simulink model "AEB_Final_PID"  (R2024b)
settings: Solver=VariableStepAuto  StartTime=0.0  StopTime=4  RelTol=1e-3
libraries: slpidlib x1, simulink x1
settings Model: Creator=garvi  LastModifiedBy=garvi
settings SolverCC: ZeroCrossControl=DisableAll

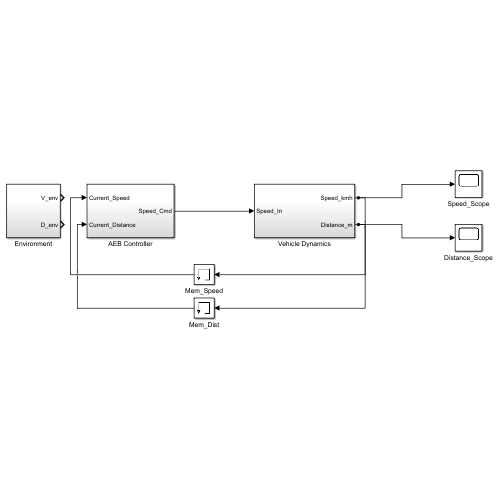
[thumbnail: Simulink's stored preview of the top-level diagram]
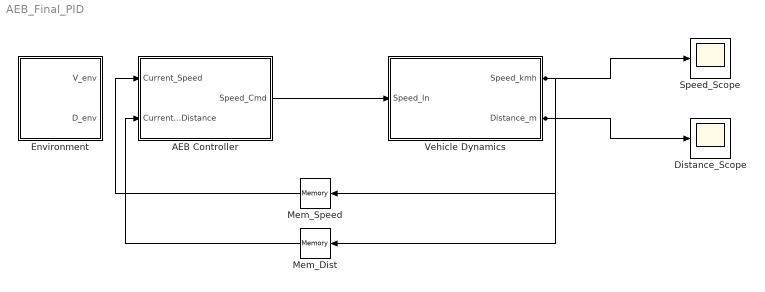
== system AEB_Final_PID ==
  AEB Controller : Subsystem
  Distance_Scope : Scope
  Environment : Subsystem
  Mem_Dist : Memory
  Mem_Speed : Memory
  Speed_Scope : Scope
  Vehicle Dynamics : Subsystem
  wires:
  AEB Controller/1(Speed_Cmd) -> Vehicle Dynamics/1(Speed_In)
  Vehicle Dynamics/1(Speed_kmh) -> Speed_Scope/1, Mem_Speed/1
  Vehicle Dynamics/2(Distance_m) -> Distance_Scope/1, Mem_Dist/1
  Mem_Speed/1 -> AEB Controller/1(Current_Speed)
  Mem_Dist/1 -> AEB Controller/2(Current_Distance)

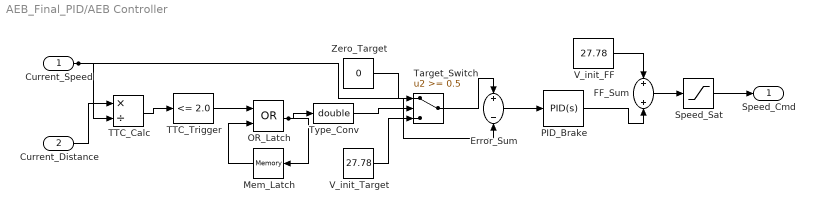
== system AEB_Final_PID/AEB Controller ==
  Current_Speed : Inport
  Current_Distance : Inport  Port=2
  Error_Sum : Sum  Inputs=+-
  FF_Sum : Sum
  Mem_Latch : Memory
  OR_Latch : Logic  Operator=OR  AllPortsSameDT=off  OutDataTypeStr=boolean
  PID_Brake : slpidlib/PID Controller  Controller=PID  Form=Parallel  TimeDomain=Continuous-time  UseExternalTs=off  SampleTime=-1  IntegratorMethod=Forward Euler  FilterMethod=Forward Euler  ControllerParametersSource=internal  P=0.1  I=0.8  UseKiTs=off  D=0  UseExternalDerivativeSource=off  N=100  UseFilter=on  TunerSelectOption=Transfer Function Based (PID Tuner App)  InitialConditionSource=internal  InitialConditionForIntegrator=0  InitialConditionForFilter=0  DifferentiatorICPrevScaledInput=0  ExternalReset=none  TrackingMode=off  Kt=1  LimitOutput=off  SatLimitsSource=internal  UpperSaturationLimit=inf  LowerSaturationLimit=-inf  LinearizeAsGain=on  AntiWindupMode=none  Kb=1  LimitIntegrator=off  UpperIntegratorSaturationLimit=inf  LowerIntegratorSaturationLimit=-inf  POutMin=[]  POutMax=[]  IOutMin=[]  IOutMax=[]  DOutMin=[]  DOutMax=[]  NOutMin=[]  NOutMax=[]  SumOutMin=[]  SumOutMax=[]  SaturationOutMin=[]  SaturationOutMax=[]  PParamMin=[]  PParamMax=[]  IParamMin=[]  IParamMax=[]  DParamMin=[]  DParamMax=[]  NParamMin=[]  NParamMax=[]  KbParamMin=[]  KbParamMax=[]  KtParamMin=[]  KtParamMax=[]  KbOutMin=[]  KbOutMax=[]  KtOutMin=[]  KtOutMax=[]  IntegratorOutMin=[]  IntegratorOutMax=[]  FilterOutMin=[]  FilterOutMax=[]  SumI1OutMin=[]  SumI1OutMax=[]  SumI2OutMin=[]  SumI2OutMax=[]  SumI3OutMin=[]  SumI3OutMax=[]  SumI4OutMin=[]  SumI4OutMax=[]  SumDOutMin=[]  SumDOutMax=[]  DifferentiatorOutMin=[]  DifferentiatorOutMax=[]  FilterDiffOutCoefMin=[]  FilterDiffOutCoefMax=[]  ReciprocalOutMin=[]  ReciprocalOutMax=[]  SumDenOutMin=[]  SumDenOutMax=[]  SumNumOutMin=[]  SumNumOutMax=[]  DivideOutMin=[]  DivideOutMax=[]  UdiffTsProdOutMin=[]  UdiffTsProdOutMax=[]  NTsProdOutMin=[]  NTsProdOutMax=[]  UintegralTsProdOutMin=[]  UintegralTsProdOutMax=[]  UngainTsProdOutMin=[]  UngainTsProdOutMax=[]  ClampingZeroOutDataTypeStr=Inherit: Inherit via back propagation  ClampingZeroOutMin=[]  ClampingZeroOutMax=[]  FilterDenConstantOutDataTypeStr=Inherit: Inherit via back propagation  FilterDenConstantOutMin=[]  FilterDenConstantOutMax=[]  PCopyOutDataTypeStr=Inherit: Inherit via back propagation  PCopyOutMin=[]  PCopyOutMax=[]  NCopyOutDataTypeStr=Inherit: Inherit via back propagation  NCopyOutMin=[]  NCopyOutMax=[]  IntegratorContinuousStateAttributes=''  IntegratorStateMustResolveToSignalObject=off  IntegratorRTWStateStorageClass=Auto  FilterContinuousStateAttributes=''  FilterStateMustResolveToSignalObject=off  FilterRTWStateStorageClass=Auto  ParallelPVariant=InternalParameters  IdealPVariant=Disabled  IVariant=InternalParameters  DVariant=InternalParameters  IntegratorVariant=Continuous  SatVariant=Disabled  AWVariant=Passthrough  PCopyVariant=Disabled  TRVariant=Disabled  FdbkBlocksVariant=Forward  IdealPFdbkVariant=Disabled  SatFdbkVariant=Disabled  DerivativeFilterVariant=ContFilter  NVariant=InternalParameters  NCopyVariant=Disabled  FilterICVariant=InternalICsFilter  IntegratorICVariant=InternalICs  ExternalResetVariant=Disabled  TRSumVariant=Passthrough  SumFdbkVariant=Disabled  SumVariant=Sum_PID  TsampFilterVariant=InternalTs  TsampNgainVariant=Passthrough  TsampIntegralVariant=Disabled_SignalSpec  ExternalSaturationOutDataTypeStr=Inherit: Same as second input  DerivativeSourceVariant=ErrorSignal  PreIntVariant=InternalPreInt
  Speed_Sat : Saturate  UpperLimit=27.78  LowerLimit=0
  TTC_Calc : Product  Inputs=*/
  TTC_Trigger : simulink/Logic and Bit Operations/Compare To Constant  relop=<=  const=2.0  OutDataTypeStr=boolean
  Target_Switch : Switch  Threshold=0.5  SaturateOnIntegerOverflow=off  InputSameDT=off
  Type_Conv : DataTypeConversion  OutDataTypeStr=double  SaturateOnIntegerOverflow=off  RndMeth=Floor
  V_init_FF : Constant  Value=27.78
  V_init_Target : Constant  Value=27.78
  Zero_Target : Constant  Value=0
  Speed_Cmd : Outport
  wires:
  Current_Distance/1 -> TTC_Calc/1
  Current_Speed/1 -> TTC_Calc/2, Error_Sum/2
  TTC_Calc/1 -> TTC_Trigger/1
  TTC_Trigger/1 -> OR_Latch/1
  Mem_Latch/1 -> OR_Latch/2
  OR_Latch/1 -> Mem_Latch/1, Type_Conv/1
  Zero_Target/1 -> Target_Switch/1
  Type_Conv/1 -> Target_Switch/2
  V_init_Target/1 -> Target_Switch/3
  Target_Switch/1 -> Error_Sum/1
  Error_Sum/1 -> PID_Brake/1
  V_init_FF/1 -> FF_Sum/1
  PID_Brake/1 -> FF_Sum/2
  FF_Sum/1 -> Speed_Sat/1
  Speed_Sat/1 -> Speed_Cmd/1

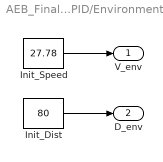
== system AEB_Final_PID/Environment ==
  Init_Dist : Constant  Value=80
  Init_Speed : Constant  Value=27.78
  V_env : Outport
  D_env : Outport  Port=2
  wires:
  Init_Speed/1 -> V_env/1
  Init_Dist/1 -> D_env/1

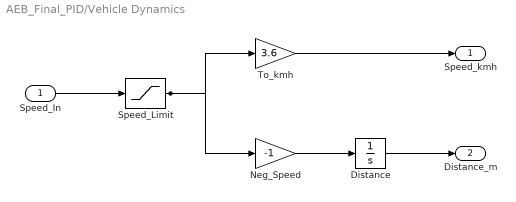
== system AEB_Final_PID/Vehicle Dynamics ==
  Speed_In : Inport
  Distance : Integrator  InitialCondition=80  LimitOutput=on  LowerSaturationLimit=0
  Neg_Speed : Gain  Gain=-1
  Speed_Limit : Saturate  UpperLimit=27.78  LowerLimit=0
  To_kmh : Gain  Gain=3.6
  Speed_kmh : Outport
  Distance_m : Outport  Port=2
  wires:
  Speed_In/1 -> Speed_Limit/1
  Speed_Limit/1 -> To_kmh/1, Neg_Speed/1
  Neg_Speed/1 -> Distance/1
  To_kmh/1 -> Speed_kmh/1
  Distance/1 -> Distance_m/1
